simulink model "AGR_WHOLESIM"  (R2022a)
settings: Solver=FixedStepDiscrete  StartTime=0.0  StopTime=1  FixedStep=0.04  RelTol=1e-3
PreLoadFcn:
  | listing = dir;
  | if (contains([listing .name], 'AGR')) && (contains([listing .name], 'MAP'))
  |     addpath('./AGR', './TRN', './FTG', './DYN', './FLCC', './GPS', './RALT', './INS', './MAP');
  | elseif (contains([listing .name], 'AGR_WHOLESIM.slx'))
  |     addpath('../AGR', '../TRN', '../FTG', '../DYN', '../FLCC', '../GPS', '../RALT', '../INS', '../MAP');
  | else
  | 
  | end
  | 
  | load('BUS_STRUCTURE_DYN.mat');
  | load('BUS_STRUCTURE_FLCC.mat');
  | load('BUS_STRUCTURE_RALT.mat');
  | load('BUS_STRUCTURE_INS.mat');
  | load('BUS_STRUCTURE_GPS.mat');
  | load('BusStructureTRN.mat');
  | load('BusStructureLOSR.mat');
  | load('BusStructureHR.mat');
  | load('BusStructureCR.mat');
  | FTG_initState;
InitFcn:
  | listing = dir;
  | if (contains([listing .name], 'TPF')) && (contains([listing .name], 'MAP'))
  |     addpath('./AGR', './TRN', './FTG', './DYN', './FLCC', './GPS', './RALT', './INS', './MAP');
  | elseif (contains([listing .name], 'AGR_WHOLESIM.slx'))
  |     addpath('../AGR', '../TRN', '../FTG', '../DYN', '../FLCC', '../GPS', '../RALT', '../INS', '../MAP');
  | else
  | 
  | end
  | 
  | load('BUS_STRUCTURE_DYN.mat');
  | load('BUS_STRUCTURE_FLCC.mat');
  | load('BUS_STRUCTURE_RALT.mat');
  | load('BUS_STRUCTURE_INS.mat');
  | load('BUS_STRUCTURE_GPS.mat');
  | load('BusStructureTRN.mat');
  | load('BusStructureLOSR.mat');
  | load('BusStructureHR.mat');
  | load('BusStructureCR.mat');
  | FTG_initState;
settings Model: Creator=ASCL  LastModifiedBy=ASCL
settings SolverCC: PositivePriorityOrder=on
settings DataIOCC: ExternalInput=[],FTGScenario.getElement('IN_TF'),FTGScenario.getElement('IN_GCAS'),FTGScenario.getElement('IN_FLIGHT_CMD')  LoadExternalInput=on  SaveOutput=off  DSMLogging=off  ReturnWorkspaceOutputs=off
settings OptimizationCC: BlockReduction=off  DefaultParameterBehavior=Inlined  UseDivisionForNetSlopeComputation=on  GainParamInheritBuiltInType=on  UseFloatMulNetSlope=on  ExpressionFolding=off  PassReuseOutputArgsAs=Individual arguments  ZeroExternalMemoryAtStartup=off  ZeroInternalMemoryAtStartup=off  EfficientFloat2IntCast=on  LifeSpan=inf  OptimizeBlockOrder=speed  DifferentSizesBufferReuse=on  EfficientTunableParamExpr=on
settings DebuggingCC: SignalInfNanChecking=warning  ReadBeforeWriteMsg=EnableAllAsError  WriteAfterWriteMsg=EnableAllAsError  WriteAfterReadMsg=EnableAllAsError  IntegerOverflowMsg=error  ParameterTunabilityLossMsg=error  UniqueDataStoreMsg=error  AssertControl=DisableAll  NonBusSignalsTreatedAsBus=error  SFInvalidInputDataAccessInChartInitDiag=error  SFTransitionOutsideNaturalParentDiag=error  SFUnreachableExecutionPathDiag=error  SFUndirectedBroadcastEventsDiag=error  IntegerSaturationMsg=error
settings HardwareCC: ProdBitPerPointer=32  ProdBitPerSizeT=32  ProdBitPerPtrDiffT=32  ProdLargestAtomicInteger=Long  ProdLargestAtomicFloat=Double  ProdEndianess=BigEndian  ProdWordSize=32  ProdLongLongMode=on  ProdHWDeviceType=Freescale->MPC83xx
settings ModelReferenceCC: ModelReferenceNumInstancesAllowed=Single
settings SFSimCC: SimCustomHeaderCode="#include \"MAP.h\""  SimUserSources=MAP.c  SimUserLibraries=WS2_32.LIB  CompileTimeRecursionLimit=0  EnableRuntimeRecursion=off  MATLABDynamicMemAlloc=off
settings RTWCC: SystemTargetFile=ert.tlc  TemplateMakefile=ert_default_tmf  GenerateReport=on  RTWUseSimCustomCode=on  CustomHeaderCode="#include \"MAP.h\""  CustomSource=MAP.c  CustomLibrary=WS2_32.LIB  BuildConfiguration=Faster Runs  IncludeHyperlinkInReport=on  LaunchReport=on  GenerateTraceInfo=on  GenerateTraceReport=on  GenerateTraceReportSl=on  GenerateTraceReportSf=on  GenerateTraceReportEml=on
settings CodeAppCC: ForceParamTrailComments=on  IgnoreCustomStorageClasses=off  OperatorAnnotations=on  SimulinkDataObjDesc=on  SFDataObjDesc=on  MATLABFcnDesc=on  InsertBlockDesc=on  StateflowObjectComments=on  MATLABSourceComments=on  EnableCustomComments=on  InlinedPrmAccess=Macros  ReqsInCode=on
settings ERTTargetCC: TargetLangStandard=C99 (ISO)  UtilityFuncGeneration=Shared location  GenerateSampleERTMain=on  IncludeMdlTerminateFcn=off  CombineSignalStateStructs=on  SuppressErrorStatus=on  SupportAbsoluteTime=off  SupportNonFinite=off  SupportComplex=off  SupportVariableSizeSignals=on  ParenthesesLevel=Standards  CastingMode=Standards  GenerateSharedConstants=off  InlinedParameterPlacement=NonHierarchical  ERTCustomFileTemplate=example_file_process.tlc  RateTransitionBlockCode=Function  PreserveIfCondition=on  ConvertIfToSwitch=off  EnableSignedLeftShifts=off  EnableSignedRightShifts=off

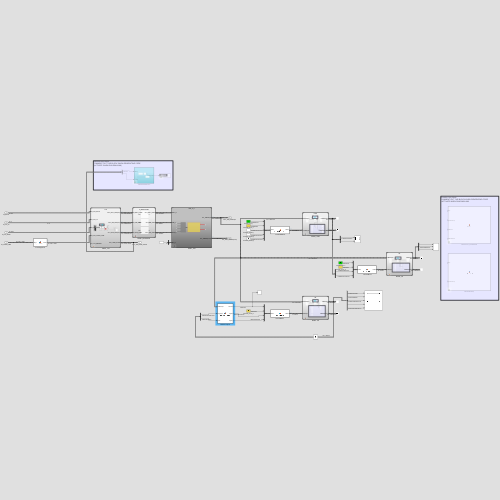
[thumbnail: Simulink's stored preview of the top-level diagram]
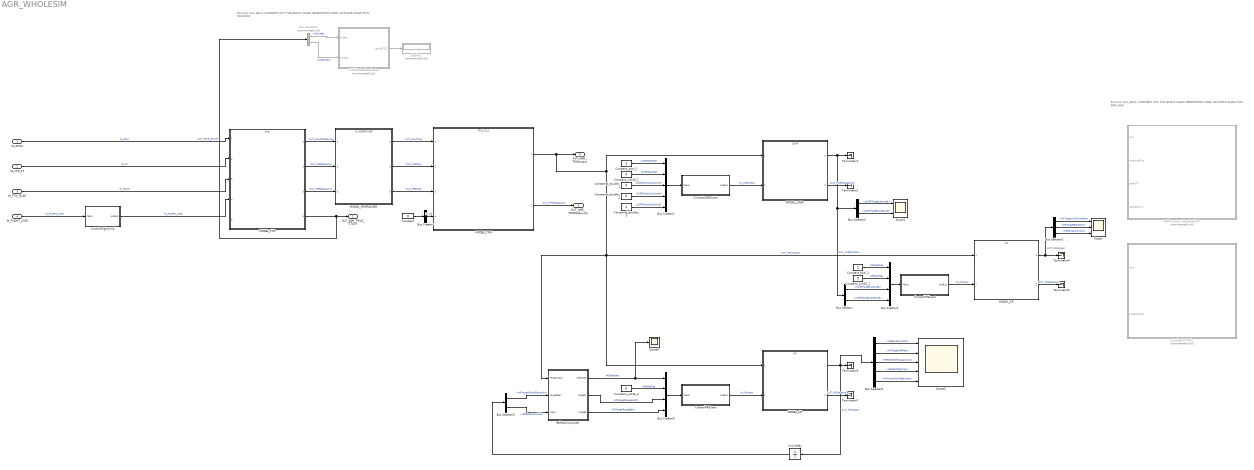
== system AGR_WHOLESIM ==
  note: Simulink Only Block
      | COMMENT OUT THIS BLOCK WHEN GENERATING CODE
      | (ACTIVATE WHEN RUN SIMULINK)
  note: Simulink Only Block
      | COMMENT OUT THIS BLOCK WHEN GENERATING CODE
      | (ACTIVATE WHEN RUN SIMULINK)
  IN_STICK : Inport  OutDataTypeStr=Bus: BUS_FLCC_STICK  BusOutputAsStruct=on
  IN_FTG_TF : Inport  Port=2  OutDataTypeStr=Bus: BUS_FLCC_TF_CMD  BusOutputAsStruct=on
  IN_FTG_GCAS : Inport  Port=3  OutDataTypeStr=Bus: BUS_FLCC_GCAS_CMD  BusOutputAsStruct=on
  IN_FLIGHT_CMD : Inport  Port=4  OutDataTypeStr=Bus: BUS_FLCC_FLIGHT_CMD  BusOutputAsStruct=on
  BallisticComputer : MATLAB Function  TreatAsAtomicUnit=on
  Bus Creator : BusCreator  Inputs=1  OutDataTypeStr=Bus: TRN_MC  NonVirtualBus=on
  Bus Creator1 : BusCreator  Inputs=5  OutDataTypeStr=Bus: LOSRInput  NonVirtualBus=on
      settings: InheritFromInputs=off
  Bus Creator2 : BusCreator  Inputs=4  OutDataTypeStr=Bus: CRInput  NonVirtualBus=on
      settings: InheritFromInputs=off
  Bus Creator3 : BusCreator  Inputs=4  OutDataTypeStr=Bus: HRInput  NonVirtualBus=on
      settings: InheritFromInputs=off
  Bus Selector : BusSelector  OutputSignals=LOSRTargetLatitude,LOSRTargetLongitude
  Bus Selector1 : BusSelector  OutputSignals=CRTargetLOSAvailable,CRTargetElevation,CRElevationValid
  Bus Selector2 : BusSelector  OutputSignals=LOSRTargetLatitude,LOSRTargetLongitude
  Bus Selector3 : BusSelector  OutputSignals=HRImpactPointElevation,HRElevationValid
  Bus Selector4 : BusSelector  Commented=on  OutputSignals=latitude,longitude
  Bus Selector5 : BusSelector  OutputSignals=HRElevationValid,HRTargetOffMap,HRSelectedWraparound,HRDataTagWrap,HRImpactPointElevation
  Constant : Constant  Value=0  OutDataTypeStr=boolean
  Constant_bool_1 : Constant  OutDataTypeStr=boolean
  Constant_bool_2 : Constant  OutDataTypeStr=boolean
  Constant_uint16_1 : Constant  Value=0  OutDataTypeStr=uint16
  Constant_uint16_2 : Constant  Value=0  OutDataTypeStr=uint16
  Constant_uint16_3 : Constant  Value=0  OutDataTypeStr=uint16
  Constantd_double_1 : Constant  Value=0  OutDataTypeStr=double
  Constantd_double_2 : Constant  Value=0  OutDataTypeStr=double
  Constantd_double_3 : Constant  OutDataTypeStr=double
  ControlCREvent : MATLAB Function  TreatAsAtomicUnit=on
  ControlFlightCmd : MATLAB Function  TreatAsAtomicUnit=on
  ControlHREvent : MATLAB Function  TreatAsAtomicUnit=on
  ControlLOSREvent : MATLAB Function  TreatAsAtomicUnit=on
  Display1 : Display  Commented=on
  InitNUpdateMapCache : Subsystem  Commented=on  TreatAsAtomicUnit=on
  MATFunction_VisualizeWCP : MATLAB Function  Commented=on  TreatAsAtomicUnit=on
  MODEL_CR : ModelReference  ModelNameDialog=CR.slx  SimulationMode=Normal  ModelReferenceVersion=1.236
  MODEL_FTG : ModelReference  ModelNameDialog=FTG.slx  SimulationMode=Normal  ModelReferenceVersion=1.456
  MODEL_HR : ModelReference  ModelNameDialog=HR.slx  SimulationMode=Normal  ModelReferenceVersion=1.371
  MODEL_LOSR : ModelReference  ModelNameDialog=LOSR.slx  SimulationMode=Normal  ModelReferenceVersion=1.330
  MODEL_MSGPACKER : ModelReference  ModelNameDialog=M_MSGPACKER.slx  SimulationMode=Normal  ModelReferenceVersion=1.294
  MODEL_TRN : ModelReference  ModelNameDialog=TRN_V3_2.slx  SimulationMode=Normal  ModelReferenceVersion=2.342
  Scope : Scope  NumInputPorts=3
  Scope1 : Scope  NumInputPorts=2
  Scope3 : Scope  NumInputPorts=5
  Scope4 : Scope
  Terminator{1..2,4..7} (6 alike) : Terminator
  Unit Delay : UnitDelay  SampleTime=-1  HasFrameUpgradeWarning=on
  VisualizeWTPOnly : MATLAB Function  Commented=on  TreatAsAtomicUnit=on
  OUT_AGR_TRUE_STATE : Outport  OutDataTypeStr=Bus: BUS_DYN_STATE  BusOutputAsStruct=on
  OUT_AGR_TRNOutput : Outport  Port=2  OutDataTypeStr=Bus: TRNOutput  BusOutputAsStruct=on
  OUT_AGR_TRNDatapump : Outport  Port=3  OutDataTypeStr=Bus: TRNDatapump
  wires:
  Bus Creator/1 -> MODEL_TRN/4  "IN_MC"
  MODEL_FTG/3 -> MODEL_MSGPACKER/3  "OUT_GPSDatapump"
  MODEL_TRN/1 -> MODEL_CR/1, BallisticComputer/1(TRNOutput), MODEL_HR/1, MODEL_LOSR/1, OUT_AGR_TRNOutput/1  "OUT_TRNOutput"
  MODEL_TRN/2 -> OUT_AGR_TRNDatapump/1  "OUT_TRNDatapump"
  Constant/1 -> Bus Creator/1
  IN_FLIGHT_CMD/1 -> ControlFlightCmd/1(inBus)  "IN_FLIGHT_CMD"
  MODEL_FTG/4 -> Bus Selector4/1, OUT_AGR_TRUE_STATE/1  "OUT_TRUE_STATE"
  Bus Selector4/2 -> InitNUpdateMapCache/2(lonDeg)  "<longitude>"
  MODEL_FTG/2 -> MODEL_MSGPACKER/2  "OUT_INSDatapump"
  IN_FTG_GCAS/1 -> MODEL_FTG/3  "IN_GCAS"
  IN_FTG_TF/1 -> MODEL_FTG/2  "IN_TF"
  MODEL_FTG/1 -> MODEL_MSGPACKER/1  "OUT_RALTDatapump"
  Bus Selector4/1 -> InitNUpdateMapCache/1(latDeg)  "<latitude>"
  IN_STICK/1 -> MODEL_FTG/1  "IN_Stick"
  ControlFlightCmd/1(outBus) -> MODEL_FTG/4  "IN_FLIGHT_CMD"
  MODEL_LOSR/1 -> Terminator1/1, Bus Selector/1, Bus Selector2/1  "OUT_LOSROutput"
  MODEL_LOSR/2 -> Terminator2/1  "OUT_LOSRDatapump"
  MODEL_CR/1 -> Bus Selector1/1, Terminator4/1  "OUT_CROutput"
  MODEL_CR/2 -> Terminator5/1  "OUT_CRDatapump"
  MODEL_HR/1 -> Bus Selector5/1, Unit Delay/1, Terminator6/1  "OUT_HROutput"
  MODEL_HR/2 -> Terminator7/1  "OUT_HRDatapump"
  Constant_uint16_1/1 -> Bus Creator1/2  "LOSRDataTag"
  Constant_bool_1/1 -> Bus Creator1/1  "LOSRSelected"
  Constantd_double_2/1 -> Bus Creator1/4  "LOSRDirectionCosineY"
  Constantd_double_1/1 -> Bus Creator1/3  "LOSRDirectionCosineX"
  Constantd_double_3/1 -> Bus Creator1/5  "LOSRDirectionCosineZ"
  Bus Selector/2 -> Bus Creator2/4  "<LOSRTargetLongitude>"
  Bus Selector/1 -> Bus Creator2/3  "<LOSRTargetLatitude>"
  Constant_uint16_2/1 -> Bus Creator2/2  "CRDataTag"
  Constant_bool_2/1 -> Bus Creator2/1  "CRSelected"
  BallisticComputer/1(selected) -> Scope4/1, Bus Creator3/1  "HRSelected"
  Constant_uint16_3/1 -> Bus Creator3/2  "HRDataTag"
  BallisticComputer/3(rangeE) -> Bus Creator3/4  "HRTargetRangeEast"
  Bus Selector1/1 -> Scope/1  "<CRTargetLOSAvailable>"
  Bus Selector1/2 -> Scope/2  "<CRTargetElevation>"
  Bus Selector1/3 -> Scope/3  "<CRElevationValid>"
  Bus Selector2/1 -> Scope1/1  "<LOSRTargetLatitude>"
  Bus Selector2/2 -> Scope1/2  "<LOSRTargetLongitude>"
  Bus Creator2/1 -> ControlCREvent/1(inBus)
  Bus Creator1/1 -> ControlLOSREvent/1(inBus)
  ControlLOSREvent/1(outBus) -> MODEL_LOSR/2  "IN_LOSRInput"
  ControlHREvent/1(outBus) -> MODEL_HR/2  "IN_HRInput"
  Bus Creator3/1 -> ControlHREvent/1(inBus)
  ControlCREvent/1(outBus) -> MODEL_CR/2  "IN_CRInput"
  Bus Selector3/1 -> BallisticComputer/2(targetElev)  "<HRImpactPointElevation>"
  Bus Selector3/2 -> BallisticComputer/3(Valid)  "<HRElevationValid>"
  Unit Delay/1 -> Bus Selector3/1
  BallisticComputer/2(rangeN) -> Bus Creator3/3  "HRTargetRangeNorth"
  Bus Selector5/5 -> Scope3/5  "<HRImpactPointElevation>"
  Bus Selector5/4 -> Scope3/4  "<HRDataTagWrap>"
  Bus Selector5/3 -> Scope3/3  "<HRSelectedWraparound>"
  Bus Selector5/2 -> Scope3/2  "<HRTargetOffMap>"
  Bus Selector5/1 -> Scope3/1  "<HRElevationValid>"
  MODEL_MSGPACKER/1 -> MODEL_TRN/1  "OUT_RALTMsg"
  MODEL_MSGPACKER/2 -> MODEL_TRN/2  "OUT_INSMsg"
  MODEL_MSGPACKER/3 -> MODEL_TRN/3  "OUT_GPSMsg"
  InitNUpdateMapCache/1(resultDTED) -> Display1/1

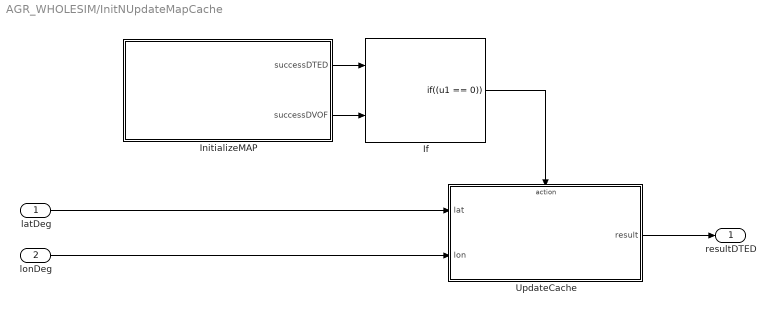
== system AGR_WHOLESIM/InitNUpdateMapCache ==
  latDeg : Inport  OutDataTypeStr=double
  lonDeg : Inport  Port=2  OutDataTypeStr=double
  If : If  NumInputs=2  IfExpression=(u1 == 0)  ShowElse=off
  InitializeMAP : MATLAB Function  TreatAsAtomicUnit=on
  UpdateCache : Subsystem  TreatAsAtomicUnit=on
  resultDTED : Outport  VectorParamsAs1DForOutWhenUnconnected=off
  wires:
  lonDeg/1 -> UpdateCache/2(lon)
  UpdateCache/1(result) -> resultDTED/1
  InitializeMAP/1(successDTED) -> If/1
  latDeg/1 -> UpdateCache/1(lat)
  InitializeMAP/2(successDVOF) -> If/2
  If/1 -> UpdateCache/Action

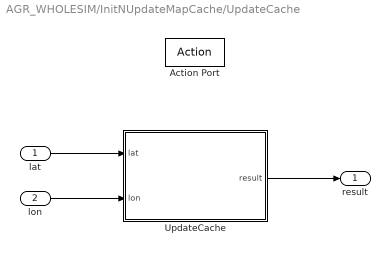
== system AGR_WHOLESIM/InitNUpdateMapCache/UpdateCache ==
  lat : Inport
  lon : Inport  Port=2
  Action Port : ActionPort  ActionPortLabel=if((u1 == 0))
  UpdateCache : MATLAB Function  TreatAsAtomicUnit=on
  result : Outport  VectorParamsAs1DForOutWhenUnconnected=off
  wires:
  UpdateCache/1(result) -> result/1
  lat/1 -> UpdateCache/1(lat)
  lon/1 -> UpdateCache/2(lon)

== matlab function AGR_WHOLESIM/InitNUpdateMapCache/InitializeMAP ==
  data: successDTED output; successDVOF output
function [successDTED, successDVOF] = InitializeMAP()
%InitializeMAP

% Persistent variable
persistent firstRun
if isempty(firstRun)
    firstRun = true;
end

% Initialize output
flagDTED = int32(1);
flagDVOF = int32(1);
successDTED = int32(1);
successDVOF = int32(1);

if firstRun
    % Path of DTED data
    pathDTED = 'C:\Users\ASCL\Documents\GitHub\DTNS\MAP\MAP_DB';

    % Length of DETD data path
    strLenDTED = int32(strlength(pathDTED));
    
    % Call [ InitialMap ] : 맵 폴더 위치 설정
    flagDTED = coder.ceval('InitialMap', pathDTED, strLenDTED );
    
    successDTED = flagDTED;

    if (successDTED)
        firstRun = false;
    end
else
    successDTED = int32(0);
    successDVOF = int32(0);
end

== matlab function AGR_WHOLESIM/MATFunction_VisualizeWCP ==
  data: wtp input; predictedTraj input; pathDTF input; pathGCAWS input
function Visualize(wtp, predictedTraj, pathDTF, pathGCAWS)
%VISUALIZE
% 
persistent fHandle subPlot1 subPlot2 tSpanWCP tSpanPT count map ARCSEC2DEG mapSurf predBound yAxisMax

acXY = zeros(2,27);
heading = 0;

% Initialize Figure Handle
if isempty(fHandle)
    fHandle = figure('WindowStyle', 'docked');
end

% Divide and Initailize the Figure
if isempty(subPlot1)
    set(0, 'CurrentFigure', fHandle);
    subPlot1 = subplot(1, 4, 1:2);
    axis equal;
    colormap(fliplr(hsv));
    view(0, 90);
    set(gca, 'Color', [0.3, 0.3, 0.3]);
    xlabel('Longitude [deg]');
    ylabel('Latitude [deg]');
    hold off;
end

% Divide and Initailize the Figure
if isempty(subPlot2)
    subPlot2 = subplot(1, 4, 3:4);
    hold on;
    grid minor;
    xlabel('Time [sec]');
    ylabel('Height [m]');
    axis([-0.5, 20, 0, 2000]);
    hold off;
end

% Initialize tSpanWCP
if isempty(tSpanWCP)
    tSpanWCP = 0:0.5:((length(wtp)-1)*0.5);
end

% Initialize tSpanPT
if isempty(tSpanPT)
    tSpanPT = 0:0.25:((size(predictedTraj, 1)-1)*0.25);
end

% Initialize count
if isempty(count)
    count = 0;    
end

% Initialize yAxisMax
if isempty(yAxisMax) 
    yAxisMax = 2000;
end
% Initialize ARCSEC2DEG
if isempty(ARCSEC2DEG)
    ARCSEC2DEG = (0.000277777777777777);
end

% Initialize map
if isempty(map)
    map = ones(150, 150, 3);

    % Current A/C Position
    latTrue = predictedTraj(1, 1, 1);
    lonTrue = predictedTraj(1, 1, 2);
    
    % Flooring to neighboring Map Grid
    latTrun = floor(latTrue/(3*ARCSEC2DEG)) * (3*ARCSEC2DEG);
    lonTrun = floor(lonTrue/(3*ARCSEC2DEG)) * (3*ARCSEC2DEG);
    
    mapSizeLat = size(map, 1);
    mapSizeLon = size(map, 2);
    % Update map data
    for ii = 1:size(map, 1)
    
        for jj = 1:size(map, 2)
            
            map(ii, jj, 1) = latTrun + (9*ARCSEC2DEG) * ((size(map, 1) - floor(mapSizeLat * 1.5)) + ii);
            map(ii, jj, 2) = lonTrun + (9*ARCSEC2DEG) * ((size(map, 2) - floor(mapSizeLon * 1.5)) + jj);
            
            map(ii, jj, 3) = ...
            coder.ceval('MAPGetTerrainHeight', map(ii, jj, 1), map(ii, jj, 2)); 

            if (ii == size(map, 1)) && (jj == size(map, 2))
                map(ii, jj, 3) = 2200;
            end
            
        end
    
    end
    
end

% Initialize mapSurf: mapSurf plot handle
if isempty(mapSurf)
    set(0, 'CurrentFigure', fHandle);
    subplot(subPlot1);
    hold on;
    mapSurf = surf(map(:,:,2), map(:,:,1), map(:,:,3), 'FaceAlpha', 0.75);
    drawnow;
    hold off;
end

% Initialize predBound: predBound plot handle
if isempty(predBound)
    set(0, 'CurrentFigure', fHandle);
    subplot(subPlot1);
    hold on;
    predBound = plot3([predictedTraj(:,2,2); flipud(predictedTraj(:,3,2))], ...
        [predictedTraj(:,2,1); flipud(predictedTraj(:,3,1))], ...
        [predictedTraj(:,2,3); flipud(predictedTraj(:,3,3))], '-m', 'LineWidth', 3);
    hold off;
end


%%

% Limit & Reset count
if (count >= 250)
    count = 0;
end

% 0.5Hz Event
if rem(count, 50) == 0
    set(0, 'CurrentFigure', fHandle);
    subplot(subPlot1);
    hold on;
    
    % Current A/C Position
    latTrue = predictedTraj(1, 1, 1);
    lonTrue = predictedTraj(1, 1, 2);
    
    % Flooring to neighboring Map Grid
    latTrun = floor(latTrue/(3*ARCSEC2DEG)) * (3*ARCSEC2DEG);
    lonTrun = floor(lonTrue/(3*ARCSEC2DEG)) * (3*ARCSEC2DEG);
    
    mapSizeLat = size(map, 1);
    mapSizeLon = size(map, 2);
    if abs(latTrun-(map(1, 1, 1)+map(end, 1, 1))/2) >= 100*(3*ARCSEC2DEG) || abs(lonTrun-(map(1, 1, 2)+map(1, end, 2))/2) >= 100*(3*ARCSEC2DEG)
        % Update map data
        for ii = 1:size(map, 1)
            for jj = 1:size(map, 2)
                map(ii, jj, 1) = latTrun + (9*ARCSEC2DEG) * ((size(map, 1) - floor(mapSizeLat * 1.5)) + ii);
                map(ii, jj, 2) = lonTrun + (9*ARCSEC2DEG) * ((size(map, 2) - floor(mapSizeLon * 1.5)) + jj);
                map(ii, jj, 3) = ...
                coder.ceval('MAPGetTerrainHeight', map(ii, jj, 1), map(ii, jj, 2)); 
            end
        end
        
        set(mapSurf, 'XData', map(:,:,2), 'YData', map(:,:,1), 'ZData', map(:,:,3));
        drawnow;
    end
    
    % Draw Map
    axis([lonTrun - (3*ARCSEC2DEG)*60, lonTrun + (3*ARCSEC2DEG)*60, latTrun - (3*ARCSEC2DEG)*60, latTrun + (3*ARCSEC2DEG)*60]);
    drawnow;
    hold off;
    
end

% 2.5Hz Event
if rem(count, 5) == 0
    set(0, 'CurrentFigure', fHandle);
    subplot(subPlot1);
    
    hold on;
    latTrue = predictedTraj(1, 1, 1);
    lonTrue = predictedTraj(1, 1, 2);
    heading = getHeadingFromVector([latTrue, lonTrue], [predictedTraj(81, 1, 1), predictedTraj(81, 1, 2)]);
    acXY = drawAircraft( [lonTrue;latTrue], 4.5*ARCSEC2DEG, heading);
    plot3(acXY(1,:), acXY(2,:), predictedTraj(1, 1, 3)*ones(size(acXY(1,:))), '-r')
    
    set(predBound, 'XData', [predictedTraj(:,2,2); flipud(predictedTraj(:,3,2))], ...
    'YData', [predictedTraj(:,2,1); flipud(predictedTraj(:,3,1))], ...
    'ZData', [predictedTraj(:,2,3); flipud(predictedTraj(:,3,3))]);
    
    hold off;
    
    set(0, 'CurrentFigure', fHandle);
    subplot(subPlot2);
    
    nominalTerrain = zeros(size(predictedTraj, 1), 1);
    for nn = 1:size(predictedTraj(:,1,3), 1)
        nominalTerrain(nn) = coder.ceval('MAPGetTerrainHeight', predictedTraj(nn, 1, 1), predictedTraj(nn, 1, 2)); 
    end
    
    hold on;
    cla
    plot(tSpanPT, nominalTerrain, '-g', 'LineWidth', 5, 'DisplayName', 'Nominal Terrain');
    plot(tSpanWCP, wtp, '-b', 'LineWidth', 5, 'DisplayName', 'WCP');
    plot(tSpanPT, predictedTraj(:, 1, 3), '--k', 'LineWidth', 2, 'DisplayName', 'Predicted Nominal Trajectory');
    plot(0, predictedTraj(1, 1, 3), 'ro', 'MarkerSize', 10, 'DisplayName', 'A/C');
    plot(0:0.5:20, pathDTF, '-y', 'DisplayName','DBTF Reference Trajectory', 'LineWidth', 2);
    
    for ii = 1:12
       plot(0:0.5:20, pathGCAWS(:,ii,3));
       
    end
    
    if (predictedTraj(1, 1, 3) > yAxisMax-300)
        axis([-0.5, 20, 0, predictedTraj(1, 1, 3) + 500]);
    elseif (predictedTraj(1, 1, 3) < 1800)
        axis([-0.5, 20, 0, 2000])
    end
    % axis([-1, 20, 300, 800]);
    drawnow;
    hold off; 
    
end

% Update count
count = count + 1;

end


function [acXY] = drawAircraft(centerXY, longLength, heading)
%DRAWAircraft
    % centerXY      (2x1)
    % longLength    (1) [deg]
    % heading       (1) [deg]
    
    acXY = zeros(2, 27);
    translate = ones(2, 27);
    translate(1,:) = translate(1,:) * centerXY(1); 
    translate(2,:) = translate(2,:) * centerXY(2); 
    
    refXY = [ 0, -2, -4, -6,-16,-16,-17,-17, -4, -4, -9,-10, -4,  0,  4, 10,  9,  4,  4, 17, 17, 16, 16,  6,  4,  2,  0;...
             25, 20,  8,  0, -7, -4, -4,-14,-14,-18,-23,-26,-25,-25,-25,-26,-23,-18,-14,-14, -4, -4, -7,  0,  8, 20, 25];
    
    acXY = refXY / 50 * longLength;
    
    rot = [cosd(-heading), -sind(-heading); sind(-heading), cosd(-heading)];
    
    acXY = rot * acXY + translate;
    
end

function [heading] = getHeadingFromVector(fromLatLon, toLatLon)
%GETHEADINGFROMVECTOR
    % fromLatLon (2x1) [deg]
    % toLatLon (2x1) [deg]
    
    dLon = toLatLon(2) - fromLatLon(2);
    
    y = sind(dLon) * cosd(toLatLon(1));
    x = cosd(fromLatLon(1)) * sind(toLatLon(1)) ...
        - sind(fromLatLon(1)) * cosd(toLatLon(1)) * cosd(dLon);
    
    heading = atan2d(y, x);
    heading = rem( heading + 360, 360);

end

== matlab function AGR_WHOLESIM/ControlFlightCmd ==
  data: inBus input Bus: BUS_FLCC_FLIGHT_CMD; outBus output Bus: BUS_FLCC_FLIGHT_CMD
function outBus = ControlFlightCmd(inBus)
%ControlFlightCmd
persistent time dt
if isempty(time)
    time = 0.0;
end
if isempty(dt)
    dt = 0.04;
end

ACTIVATED = true;

% -switchGCAS
SWICH_GCAS_NOT_SELECTED = uint8(0);
SWICH_GCAS_SELECTED     = uint8(1);
SWICH_GCAS_AUTO_GCAS    = uint8(2);

% -switchTF
SWICH_TF_NOT_SELECTED   = uint8(0);
SWICH_TF_SELECTED       = uint8(1);
SWICH_TF_AUTO_TF        = uint8(2);

% -switchRoll
SWITCH_ROLL_ATT_HOLD    = uint8(0);
SWITCH_ROLL_STRG_SEL    = uint8(1);
SWITCH_ROLL_HDG_SEL     = uint8(2);

% -switchPitch
SWITCH_PITCH_AP_OFF     = uint8(0);
SWITCH_PITCH_ATT_HOLD   = uint8(1);
SWITCH_PITCH_ALT_HOLD   = uint8(2);

% Copy
outBus = inBus;

if ACTIVATED

    % [WTPG] Sim: Roll
%     outBus = SET_ATF(outBus, false, time, 0, inf);
%     outBus = SET_ROLL_ATT(outBus, 30, time, 20, 20);
%     outBus = SET_ROLL_ATT(outBus, -30, time, 40, 20);
%     outBus = SET_ROLL_ATT(outBus, 0, time, 60, inf);

    % [DTF & GCAWS] Feasibility Sim
%     outBus.switchRoll = uint8(0);
%     outBus.switchPitch = uint8(2);
%     outBus.refSpeed = SET_VALUE(outBus.refSpeed, 100, time, 0, 40);
%     outBus.refSpeed = SET_VALUE(outBus.refSpeed, 100, time, 40, 40);
%     outBus.nextAlt = 2000;
%     outBus.setRoll = 0;

%     outBus.refSpeed = 300;
%     outBus.nextLat = 45.70;
%     outBus.nextLon = 127.6;
    outBus.nextAlt = 2000.0;
end

% Update Time
time = time + dt;
end

function out = SET_ATF(in, isATF, curTime, triggerTime, duration)
% -switchTF
SWICH_TF_NOT_SELECTED   = uint8(0);
SWICH_TF_SELECTED       = uint8(1);
SWICH_TF_AUTO_TF        = uint8(2);

out = in;
if (triggerTime <= curTime) && (curTime <= triggerTime+duration)
    if isATF
        out.switchTF = SWICH_TF_AUTO_TF;
    else
        out.switchTF = SWICH_TF_SELECTED;
    end

else
end
end

function out = SET_ROLL_ATT(in, rollAngle, curTime, triggerTime, duration)
% -switchRoll
SWITCH_ROLL_ATT_HOLD    = uint8(0);
SWITCH_ROLL_STRG_SEL    = uint8(1);
SWITCH_ROLL_HDG_SEL     = uint8(2);

out = in;
if (triggerTime <= curTime) && (curTime <= triggerTime+duration)
    out.switchRoll = SWITCH_ROLL_ATT_HOLD;
    out.setRoll = rollAngle;
else
end
end

function out = SET_VALUE(in, value, curTime, triggerTime, duration)
out = in;
if (triggerTime <= curTime) && (curTime <= triggerTime+duration)
    out = value;
else
end
end

== matlab function AGR_WHOLESIM/VisualizeWTPOnly ==
  data: wtp input; predictedTraj input
function VisualizeWTPOnly(wtp, predictedTraj)
%VisualizeWTPOnly
% 
persistent fHandle subPlot1 subPlot2 tSpanWCP tSpanPT count map ARCSEC2DEG mapSurf predBound yAxisMax

acXY = zeros(2,27);
heading = 0;

% Initialize Figure Handle
if isempty(fHandle)
    fHandle = figure('WindowStyle', 'docked');
end

% Divide and Initailize the Figure
if isempty(subPlot1)
    set(0, 'CurrentFigure', fHandle);
%     subPlot1 = subplot(5, 1, 1:4, 'position', [0.05 0.525 0.9 0.425]);
    subPlot1 = subplot(1, 4, 1:2);
    axis equal;
    colormap(fliplr(hsv));
    view(0, 90);
    set(gca, 'Color', [0.3, 0.3, 0.3]);
    xlabel('Longitude [deg]');
    ylabel('Latitude [deg]');
    hold off;
end

% Divide and Initailize the Figure
if isempty(subPlot2)
%     subPlot2 = subplot(5, 1, 5, 'position', [0.1 0.05 0.8 0.425]);
    subPlot2 = subplot(1, 4, 3:4);
    hold on;
    grid minor;
    xlabel('Time [sec]');
    ylabel('Height [m]');
    axis([-0.5, 20, 0, 2000]);
    hold off;
end

% Initialize tSpanWCP
if isempty(tSpanWCP)
    tSpanWCP = 0:0.5:((length(wtp)-1)*0.5);
end

% Initialize tSpanPT
if isempty(tSpanPT)
    tSpanPT = 0:0.25:((size(predictedTraj, 1)-1)*0.25);
end

% Initialize count
if isempty(count)
    count = 0;    
end

% Initialize yAxisMax
if isempty(yAxisMax) 
    yAxisMax = 2000;
end
% Initialize ARCSEC2DEG
if isempty(ARCSEC2DEG)
    ARCSEC2DEG = (0.000277777777777777);
end

% Initialize map
if isempty(map)
    map = ones(150, 150, 3);

    % Current A/C Position
    latTrue = predictedTraj(1, 1, 1);
    lonTrue = predictedTraj(1, 1, 2);
    
    % Flooring to neighboring Map Grid
    latTrun = floor(latTrue/(3*ARCSEC2DEG)) * (3*ARCSEC2DEG);
    lonTrun = floor(lonTrue/(3*ARCSEC2DEG)) * (3*ARCSEC2DEG);
    
    mapSizeLat = size(map, 1);
    mapSizeLon = size(map, 2);
    % Update map data
    for ii = 1:size(map, 1)
    
        for jj = 1:size(map, 2)
            
            map(ii, jj, 1) = latTrun + (9*ARCSEC2DEG) * ((size(map, 1) - floor(mapSizeLat * 1.5)) + ii);
            map(ii, jj, 2) = lonTrun + (9*ARCSEC2DEG) * ((size(map, 2) - floor(mapSizeLon * 1.5)) + jj);
            
            map(ii, jj, 3) = ...
            coder.ceval('MAPGetTerrainHeight', map(ii, jj, 1), map(ii, jj, 2)); 
            if (ii == size(map, 1)) && (jj == size(map,2))
                map(ii, jj, 3) = 2000;
            end
            
        end
    
    end
    
end

% Initialize mapSurf: mapSurf plot handle
if isempty(mapSurf)
    set(0, 'CurrentFigure', fHandle);
    subplot(subPlot1);
    hold on;
    mapSurf = surf(map(:,:,2), map(:,:,1), map(:,:,3), 'FaceAlpha', 0.85);
    drawnow;
    hold off;
end

% Initialize predBound: predBound plot handle
if isempty(predBound)
    set(0, 'CurrentFigure', fHandle);
    subplot(subPlot1);
    hold on;
    predBound = plot3([predictedTraj(:,2,2); flipud(predictedTraj(:,3,2))], ...
        [predictedTraj(:,2,1); flipud(predictedTraj(:,3,1))], ...
        [predictedTraj(:,2,3); flipud(predictedTraj(:,3,3))], '-m', 'LineWidth', 3);
    hold off;
end


%%

% Limit & Reset count
if (count >= 250)
    count = 0;
end

% 5Hz Event
if rem(count, 5) == 0
    set(0, 'CurrentFigure', fHandle);
    subplot(subPlot1);
    hold on;
    
    % Current A/C Position
    latTrue = predictedTraj(1, 1, 1);
    lonTrue = predictedTraj(1, 1, 2);
    
    % Flooring to neighboring Map Grid
    latTrun = floor(latTrue/(3*ARCSEC2DEG)) * (3*ARCSEC2DEG);
    lonTrun = floor(lonTrue/(3*ARCSEC2DEG)) * (3*ARCSEC2DEG);
    
    mapSizeLat = size(map, 1);
    mapSizeLon = size(map, 2);
    if abs(latTrun-(map(1, 1, 1)+map(end, 1, 1))/2) >= 100*(3*ARCSEC2DEG) || abs(lonTrun-(map(1, 1, 2)+map(1, end, 2))/2) >= 100*(3*ARCSEC2DEG)
        % Update map data
        for ii = 1:size(map, 1)
            for jj = 1:size(map, 2)
                map(ii, jj, 1) = latTrun + (9*ARCSEC2DEG) * ((size(map, 1) - floor(mapSizeLat * 1.5)) + ii);
                map(ii, jj, 2) = lonTrun + (9*ARCSEC2DEG) * ((size(map, 2) - floor(mapSizeLon * 1.5)) + jj);
                map(ii, jj, 3) = ...
                coder.ceval('MAPGetTerrainHeight', map(ii, jj, 1), map(ii, jj, 2)); 
            end
        end
        
        set(mapSurf, 'XData', map(:,:,2), 'YData', map(:,:,1), 'ZData', map(:,:,3));
        drawnow;
    end
    
    % Draw Map
    axis([lonTrun - (3*ARCSEC2DEG)*60, lonTrun + (3*ARCSEC2DEG)*60, latTrun - (3*ARCSEC2DEG)*60, latTrun + (3*ARCSEC2DEG)*60]);
    drawnow;
    hold off;
    
end

% 2.5Hz Event
if rem(count, 5) == 0
    set(0, 'CurrentFigure', fHandle);
    subplot(subPlot1);
    
    hold on;
    latTrue = predictedTraj(1, 1, 1);
    lonTrue = predictedTraj(1, 1, 2);
    heading = getHeadingFromVector([latTrue, lonTrue], [predictedTraj(81, 1, 1), predictedTraj(81, 1, 2)]);
    acXY = drawAircraft( [lonTrue;latTrue], 4.5*ARCSEC2DEG, heading);
    plot3(acXY(1,:), acXY(2,:), predictedTraj(1, 1, 3)*ones(size(acXY(1,:))), '-r')
    
    set(predBound, 'XData', [predictedTraj(:,2,2); flipud(predictedTraj(:,3,2))], ...
    'YData', [predictedTraj(:,2,1); flipud(predictedTraj(:,3,1))], ...
    'ZData', [predictedTraj(:,2,3); flipud(predictedTraj(:,3,3))]+200);
    
    hold off;
    
    set(0, 'CurrentFigure', fHandle);
    subplot(subPlot2);
    
    nominalTerrain = zeros(size(predictedTraj, 1), 1);
    for nn = 1:size(predictedTraj(:,1,3), 1)
        nominalTerrain(nn) = coder.ceval('MAPGetTerrainHeight', predictedTraj(nn, 1, 1), predictedTraj(nn, 1, 2)); 
    end
    
    hold on;
    cla
    plot(tSpanPT, nominalTerrain, '-g', 'LineWidth', 5, 'DisplayName', 'Nominal Terrain');
    plot(tSpanWCP, wtp, '-b', 'LineWidth', 5, 'DisplayName', 'WCP');

    if (predictedTraj(1, 1, 3) > yAxisMax-300)
        axis([-0.5, 20, 0, predictedTraj(1, 1, 3) + 500]);
    elseif (predictedTraj(1, 1, 3) < 1800)
        axis([-0.5, 20, 0, 2000])
    end
    % axis([-1, 20, 300, 800]);
    drawnow;
    hold off; 
    
end

% Update count
count = count + 1;

end


function [acXY] = drawAircraft(centerXY, longLength, heading)
%DRAWAircraft
    % centerXY      (2x1)
    % longLength    (1) [deg]
    % heading       (1) [deg]
    
    acXY = zeros(2, 27);
    translate = ones(2, 27);
    translate(1,:) = translate(1,:) * centerXY(1); 
    translate(2,:) = translate(2,:) * centerXY(2); 
    
    refXY = [ 0, -2, -4, -6,-16,-16,-17,-17, -4, -4, -9,-10, -4,  0,  4, 10,  9,  4,  4, 17, 17, 16, 16,  6,  4,  2,  0;...
             25, 20,  8,  0, -7, -4, -4,-14,-14,-18,-23,-26,-25,-25,-25,-26,-23,-18,-14,-14, -4, -4, -7,  0,  8, 20, 25];
    
    acXY = refXY / 50 * longLength;
    
    rot = [cosd(-heading), -sind(-heading); sind(-heading), cosd(-heading)];
    
    acXY = rot * acXY + translate;
    
end

function [heading] = getHeadingFromVector(fromLatLon, toLatLon)
%GETHEADINGFROMVECTOR
    % fromLatLon (2x1) [deg]
    % toLatLon (2x1) [deg]
    
    dLon = toLatLon(2) - fromLatLon(2);
    
    y = sind(dLon) * cosd(toLatLon(1));
    x = cosd(fromLatLon(1)) * sind(toLatLon(1)) ...
        - sind(fromLatLon(1)) * cosd(toLatLon(1)) * cosd(dLon);
    
    heading = atan2d(y, x);
    heading = rem( heading + 360, 360);

end

== matlab function AGR_WHOLESIM/ControlLOSREvent ==
  data: outBus output Bus: LOSRInput; inBus input Bus: LOSRInput
function outBus  = ControlLOSRSimEvent(inBus)
%ControlAGREvent
persistent time dt
if isempty(time)
    time = 0.0;
end
if isempty(dt)
    dt = 0.04;
end

ACTIVATED = false;

% Copy
outBus   = inBus;

if ACTIVATED

    outBus.LOSRSelected = SET_VALUE(inBus.LOSRSelected, false, time, 35, 1);

end


time = time + dt;
end


function out = SET_VALUE(in, value, curTime, triggerTime, duration)
out = in;
if (triggerTime <= curTime) && (curTime <= triggerTime+duration)
    out = value;
else
end
end

== matlab function AGR_WHOLESIM/ControlCREvent ==
  data: outBus output Bus: CRInput; inBus input Bus: CRInput
function outBus  = ControlCREvent(inBus)
%ControlCREvent
persistent time dt
if isempty(time)
    time = 0.0;
end
if isempty(dt)
    dt = 0.04;
end

ACTIVATED = false;

% Copy
outBus   = inBus;

if ACTIVATED

%     outBus.CRSelected = SET_VALUE(inBus.CRSelected, false, time, 55, 1);

end


time = time + dt;
end


function out = SET_VALUE(in, value, curTime, triggerTime, duration)
out = in;
if (triggerTime <= curTime) && (curTime <= triggerTime+duration)
    out = value;
else
end
end

== matlab function AGR_WHOLESIM/ControlHREvent ==
  data: outBus output Bus: HRInput; inBus input Bus: HRInput
function outBus  = ControlHREvent(inBus)
%ControlHREvent
persistent time dt
if isempty(time)
    time = 0.0;
end
if isempty(dt)
    dt = 0.04;
end

ACTIVATED = false;

% Copy
outBus   = inBus;

if ACTIVATED

%     outBus.HRSelected = SET_VALUE(inBus.HRSelected, false, time, 45, 1);

end


time = time + dt;
end


function out = SET_VALUE(in, value, curTime, triggerTime, duration)
out = in;
if (triggerTime <= curTime) && (curTime <= triggerTime+duration)
    out = value;
else
end
end

== matlab function AGR_WHOLESIM/BallisticComputer ==
  data: TRNOutput input Bus: TRNOutput; selected output; rangeN output; rangeE output; targetElev input; Valid input
function [selected, rangeN, rangeE] = BallisticComputer(TRNOutput, targetElev, Valid)
%BallisticComputer

% Initialize outputs
selected = true;
rangeN = 0.0;
rangeE = 0.0;

x = 0.0;
z = 0.0;


% Rearrange variables
llh = [TRNOutput.TRNEstOfLatitude; ...
    TRNOutput.TRNEstOfLongitude; ...
    TRNOutput.Altitude_INS - TRNOutput.TRNEstOfINSAltitudeErr];

velXYZ = [TRNOutput.TRN_VelocityX; ...
    TRNOutput.TRN_VelocityY; ...
    TRNOutput.TRN_VelocityZ];

attiDeg = [TRNOutput.TRN_Roll; TRNOutput.TRN_Pitch; TRNOutput.TRN_Yaw];

if Valid
    velNED = body2ned(velXYZ, attiDeg);
    V0 = norm(velNED);
    gamma = atan2d(-velNED(3), sqrt(velNED(1)^2+velNED(2)^2));
    z0 = llh(3);
    x0 = 0;
    T = findTime(double(targetElev), z0, V0, gamma);
    if T >= 0

        heading = atan2d(velNED(2), velNED(1));
        [x, z] = bombKinematics(x0, z0, V0, gamma, T);
        selected = true;
        rangeN = x * cosd(heading);
        rangeE = x * sind(heading);
    else
        selected = false;
        rangeN = 0.0;
        rangeE = 0.0;
    end


else
    selected = true;
    rangeN = 0.0;
    rangeE = 0.0;
end

end

%% Internal functions
function [x, z] = bombKinematics(x0, z0, V0, gamma, t)
    
    g = 9.8;
    x = x0 + V0 * cosd(gamma) .* t;
    z = z0 + V0 * sind(gamma) .* t - 0.5 * g * t.^2;
end

function T = findTime(z, z0, V0, gamma)

g = 9.8;

temp = V0^2*(sind(gamma))^2 - 2*g*(z-z0);

if temp < 0
    T = 0;
else
    T = (V0*sind(gamma) + sqrt(V0^2*(sind(gamma))^2 - 2*g*(z-z0) ) ) / g;
end
end

function [state_eb_n, C_b_n] = body2ned(state_eb_b, eulerDeg)
%body2ned
% Compute the transformation from {Body} frame to local {NED} frame
%
% == Inputs =========
% state_eb_b        - states measured w.r.t. {ECEF} and resolved in {Body}
% eulerDeg          - attitude (euler angles roll-pitch-yaw seq.) [deg]
%
% == Outputs ========
% state_eb_n        - xyz-states resolved in {NED}
% C_b_n             - Transformation matirx from {Body} to {NED} (3x3)
% 

state_eb_n  = zeros(3,1);
C_b_n       = zeros(3,3);

% Body to NED
cRol = cosd(eulerDeg(1));
sRol = sind(eulerDeg(1));
cPit = cosd(eulerDeg(2));
sPit = sind(eulerDeg(2));
cYaw = cosd(eulerDeg(3));
sYaw = sind(eulerDeg(3));
% 
% C_n_b   = [              cPit*cYaw,                cPit*sYaw,     -sPit;...
%           sRol*sPit*cYaw-cRol*sYaw, sRol*sPit*sYaw+cRol*cYaw, sRol*cPit;...
%           cRol*sPit*cYaw+sRol*sYaw, cRol*sPit*sYaw-sRol*cYaw, cRol*cPit];

C_b_n   = [ cPit*cYaw, sRol*sPit*cYaw-cRol*sYaw, cRol*sPit*cYaw+sRol*sYaw;...
            cPit*sYaw, sRol*sPit*sYaw+cRol*cYaw, cRol*sPit*sYaw-sRol*cYaw;...
                -sPit,                sRol*cPit,                cRol*cPit];
% C_b_n   = C_n_b';
      
state_eb_n  = C_b_n * state_eb_b;


end

== matlab function AGR_WHOLESIM/InitNUpdateMapCache/UpdateCache/UpdateCache ==
  data: result output; lat input; lon input
function result = UpdateCache(lat, lon)
%UpdateCache

% Persistent variables
persistent latPrev lonPrev
if isempty(latPrev)
    latPrev = 0.0;
end
if isempty(lonPrev)
    lonPrev = 0.0;
end

% Initialize output
result = int32(1);

if ( abs(lat - latPrev) > 0.05 ) || ( abs(lon - lonPrev) > 0.05)
    result = coder.ceval('UpdateCache', lat, lon);
    latPrev = lat;
    lonPrev = lon;
else
    
end
